simulink model "posadka"  (Simulink 10.2)
settings: Solver=ode45  StartTime=0.0  StopTime=20.0  RelTol=1e-3  EnableMultiTasking=on
values from neighbouring files (symbols this model uses):
  a1 = 0.37    [Lab_rab_5.m]
  a2 = 5.88    [Lab_rab_5.m]
  a3 = 8.0    (= 8)    [Lab_rab_5.m]
  a4 = 1.    (= 1)    [Lab_rab_5.m]
  a5 = 0.13    [Lab_rab_5.m]
  D = input('Çàäàéòå çíà÷åíèå äàëüíîñòè D: ')    [Lab_rab_5.m]
  Kc = -a3*a4/(a1*a4+a2)    (= -1.28)    [Lab_rab_5.m]
  Keg = Kegmax/4    [Lab_rab_5.m]
  KSIc = Tc*(a1+a4+a5)/2    [Lab_rab_5.m]
  Ktet = 1.1    [Lab_rab_5.m]
  Kwz = 0.45    [Lab_rab_5.m]
  N_of_var = input('Ââåäèòå íîìåð âàðèàíòà: ')    [Lab_rab_5.m]
  T1c = 1/a4    (= 1)    [Lab_rab_5.m]
  Tc = 1/sqrt(a1*a4+a2)    [Lab_rab_5.m]
  Teg = Tau1    (= 1.82)    [Lab_rab_5.m]
  V = 90    [Lab_rab_5.m]
libraries: simulink x2
settings Model: Creator=User  LastModifiedBy=User  ExtModeTrigMode=oneshot  ExtModeArmWhenConnect=off
settings OptimizationCC: BlockReduction=off  BooleanDataType=off  LifeSpan=auto
settings DebuggingCC: SaveWithParameterizedLinksMsg=none  SignalResolutionControl=TryResolveAllWithWarning  MultiTaskDSMMsg=warning  MultiTaskCondExecSysMsg=none  FcnCallInpInsideContextMsg=error  SFUnexpectedBacktrackingDiag=error  SFNoUnconditionalDefaultTransitionDiag=error  SFExecutionAtInitializationDiag=warning  ArithmeticOperatorsInVariantConditions=error
settings HardwareCC: ProdBitPerPointer=64  ProdBitPerSizeT=64  ProdBitPerPtrDiffT=64  ProdLargestAtomicFloat=Float  ProdIntDivRoundTo=Zero  ProdEndianess=LittleEndian  ProdWordSize=64  ProdHWDeviceType=Intel->x86-64 (Windows64)  TargetUnknown=on
settings SFSimCC: SimUseLocalCustomCode=on  CustomCodeUndefinedFunction=FilterOut
settings RTWCC: RTWUseLocalCustomCode=on
settings CodeAppCC: StateflowObjectComments=off
settings GRTTargetCC: TargetLangStandard=C99 (ISO)
settings ConfigComp: CovMetricSettings=dwe  CovSaveCumulativeToWorkspaceVar=off  CovSaveSingleToWorkspaceVar=off  CovExternalEMLEnable=on

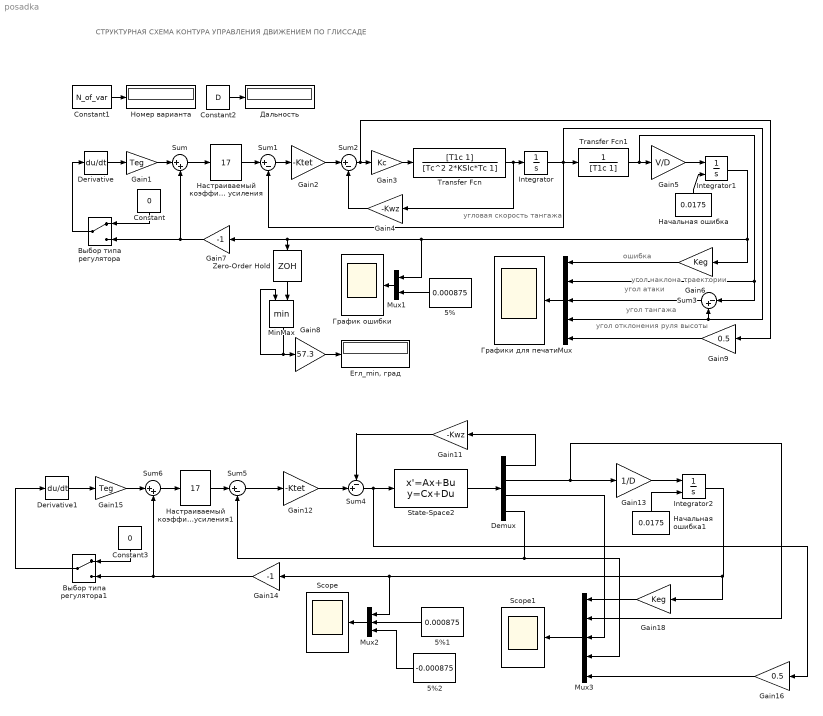
== system posadka ==
  note: СТРУКТУРНАЯ СХЕМА КОНТУРА УПРАВЛЕНИЯ ДВИЖЕНИЕМ ПО ГЛИССАДЕ
  note: ошибка
  note: угол наклона траектории
  note: угол атаки
  note: угол тангажа
  note: угол отклонения руля высоты
  note: угловая скорость тангажа
  5% : Constant  Value=0.000875
  5%1 : Constant  Value=0.000875
  5%2 : Constant  Value=-0.000875
  Constant : Constant  Value=0
  Constant1 : Constant  Value=N_of_var
  Constant2 : Constant  Value=D
  Constant3 : Constant  Value=0
  Demux : Demux
  Derivative : Derivative
  Derivative1 : Derivative
  Gain1 : Gain  Gain=Teg  SaturateOnIntegerOverflow=on
  Gain11 : Gain  Gain=-Kwz  SaturateOnIntegerOverflow=on
  Gain12 : Gain  Gain=-Ktet  SaturateOnIntegerOverflow=on
  Gain13 : Gain  Gain=1/D  SaturateOnIntegerOverflow=on
  Gain14 : Gain  Gain=-1  SaturateOnIntegerOverflow=on
  Gain15 : Gain  Gain=Teg  SaturateOnIntegerOverflow=on
  Gain16 : Gain  Gain=0.5  SaturateOnIntegerOverflow=on
  Gain18 : Gain  Gain=Keg  SaturateOnIntegerOverflow=on
  Gain2 : Gain  Gain=-Ktet  SaturateOnIntegerOverflow=on
  Gain3 : Gain  Gain=Kc  SaturateOnIntegerOverflow=on
  Gain4 : Gain  Gain=-Kwz  SaturateOnIntegerOverflow=on
  Gain5 : Gain  Gain=V/D  SaturateOnIntegerOverflow=on
  Gain6 : Gain  Gain=Keg  SaturateOnIntegerOverflow=on
  Gain7 : Gain  Gain=-1  SaturateOnIntegerOverflow=on
  Gain8 : Gain  Gain=57.3  SaturateOnIntegerOverflow=on
  Gain9 : Gain  Gain=0.5  SaturateOnIntegerOverflow=on
  Integrator : Integrator
  Integrator1 : Integrator  InitialConditionSource=external
  Integrator2 : Integrator  InitialConditionSource=external
  MinMax : MinMax  Inputs=2
  Mux : Mux  Inputs=5
  Mux1 : Mux  Inputs=2
  Mux2 : Mux  Inputs=3
  Mux3 : Mux  Inputs=5
  Scope : Scope
  Scope1 : Scope
  State-Space2 : StateSpace  A=[-(a1+a5) 0 a5*a4-a2 0;0 0 a4*V 0; 1 0 -a4 0; 1 0 0 0]  B=[-a3;0;0;0]  C=[1 0 0 0;0 1 0 0;0 0 1 0; 0 0 0 1]  D=[0;0;0;0]  InitialCondition=0
  Sum : Sum  Inputs=|++  SaturateOnIntegerOverflow=on
  Sum1 : Sum  Inputs=|+-  SaturateOnIntegerOverflow=on
  Sum2 : Sum  Inputs=|+-  SaturateOnIntegerOverflow=on
  Sum3 : Sum  Inputs=|-+  SaturateOnIntegerOverflow=on
  Sum4 : Sum  Inputs=-+|  SaturateOnIntegerOverflow=on
  Sum5 : Sum  Inputs=|+-  SaturateOnIntegerOverflow=on
  Sum6 : Sum  Inputs=|++  SaturateOnIntegerOverflow=on
  Transfer Fcn : TransferFcn  Numerator=[T1c 1]  Denominator=[Tc^2 2*KSIc*Tc 1]
  Transfer Fcn1 : TransferFcn  Denominator=[T1c 1]
  Zero-Order Hold : ZeroOrderHold
  Выбор типа регулятора : ManualSwitch
  Выбор типа регулятора1 : ManualSwitch
  График ошибки : Scope
  Графики для печати : Scope
  Дальность : Display
  "Егл_min, град" : Display
  Настраиваемый коэффициент усиления : simulink/Math Operations/Slider Gain  gain=17  low=0  high=67.5
  Настраиваемый коэффициент усиления1 : simulink/Math Operations/Slider Gain  gain=17  low=0  high=67.5
  Начальная ошибка : Constant  Value=0.0175
  Начальная ошибка1 : Constant  Value=0.0175
  Номер варианта : Display
  wires:
  Constant1/1 -> Номер варианта/1
  Constant2/1 -> Дальность/1
  Derivative/1 -> Gain1/1
  Gain1/1 -> Sum/1
  Sum/1 -> Настраиваемый коэффициент усиления/1
  Sum1/1 -> Gain2/1
  Gain2/1 -> Sum2/1
  Gain3/1 -> Transfer Fcn/1
  Transfer Fcn/1 -> Integrator/1, Gain4/1
  Gain4/1 -> Sum2/2
  Integrator/1 -> Transfer Fcn1/1, Sum1/2, Sum3/2, Mux/4
  Gain5/1 -> Integrator1/1
  Выбор типа регулятора/1 -> Derivative/1
  Constant/1 -> Выбор типа регулятора/1
  Начальная ошибка/1 -> Integrator1/2
  Transfer Fcn1/1 -> Gain5/1, Sum3/1, Mux/2
  Настраиваемый коэффициент усиления/1 -> Sum1/1
  Mux/1 -> Графики для печати/1
  Sum3/1 -> Mux/3
  Gain6/1 -> Mux/1
  Integrator1/1 -> Gain6/1, Mux1/1, Gain7/1, Zero-Order Hold/1
  Gain7/1 -> Выбор типа регулятора/2, Sum/2
  Mux1/1 -> График ошибки/1
  5%/1 -> Mux1/2
  Zero-Order Hold/1 -> MinMax/2
  MinMax/1 -> Gain8/1, MinMax/1
  Gain8/1 -> "Егл_min, град"/1
  Gain9/1 -> Mux/5
  Sum2/1 -> Gain3/1, Gain9/1
  State-Space2/1 -> Demux/1
  Sum4/1 -> State-Space2/1, Gain16/1
  Demux/1 -> Gain11/1
  Gain11/1 -> Sum4/1
  Gain12/1 -> Sum4/2
  Sum5/1 -> Gain12/1
  Demux/2 -> Mux3/2, Gain13/1
  Gain13/1 -> Integrator2/1
  Начальная ошибка1/1 -> Integrator2/2
  Sum6/1 -> Настраиваемый коэффициент усиления1/1
  Настраиваемый коэффициент усиления1/1 -> Sum5/1
  Gain14/1 -> Sum6/2, Выбор типа регулятора1/2
  Constant3/1 -> Выбор типа регулятора1/1
  Выбор типа регулятора1/1 -> Derivative1/1
  Derivative1/1 -> Gain15/1
  5%1/1 -> Mux2/2
  Mux2/1 -> Scope/1
  5%2/1 -> Mux2/3
  Mux3/1 -> Scope1/1
  Gain15/1 -> Sum6/1
  Gain16/1 -> Mux3/5
  Integrator2/1 -> Mux2/1, Gain14/1, Gain18/1
  Gain18/1 -> Mux3/1
  Demux/3 -> Mux3/3
  Demux/4 -> Mux3/4, Sum5/2
